simulink model "mpc_lateralcontrol"  (R2021a)
settings: Solver=VariableStepAuto  StartTime=0.0  StopTime=Ts  FixedStep=0.1  RelTol=1e-3
InitFcn:
  | mpc_init
StopFcn:
  | simulation_plots_mpc
values from neighbouring files (symbols this model uses):
  Vx = 25    [mpc_init.m]
libraries: mpclib x1
settings Model: Creator=anime  LastModifiedBy=User
settings SolverCC: AlgebraicLoopSolver=TrustRegion
settings DebuggingCC: SFMachineParentedDataDiag=warning

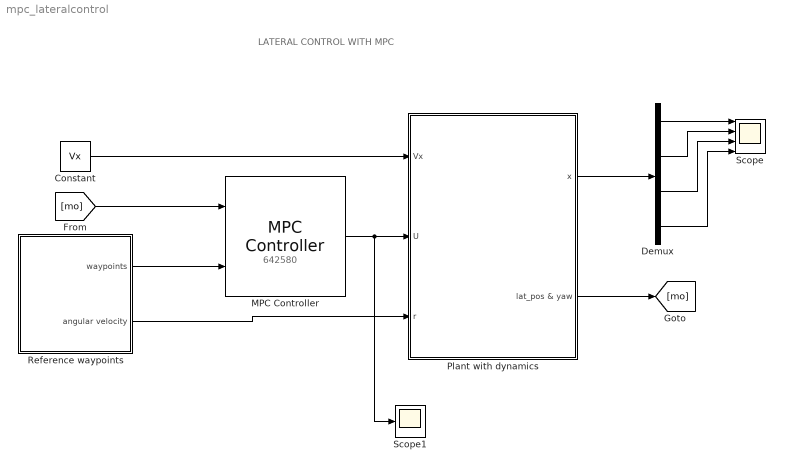
== system mpc_lateralcontrol ==
  note: 642580
  note: LATERAL CONTROL WITH MPC
  Constant : Constant  Value=Vx
  Demux : Demux
  MPC Controller : mpclib/MPC Controller  SCDEnableBlockLinearizationSpecification=on  mpcobj=mpc1  is_multiple=0  enable_value=0  return_u0=off  updateMPCinCallerWorkspace=on  md_inport=off  mv_inport=off  uref_inport=off  return_cost=off  return_mvseq=off  return_qpstatus=off  return_xseq=off  return_state=off  return_ovseq=off  state_inport=off  umin_inport=off  umax_inport=off  ymin_inport=off  ymax_inport=off  cc_inport=off  ywt_inport=off  uwt_inport=off  duwt_inport=off  rhoeps_inport=off  pm_inport=off  MaximumP=10  HorizonChoice=FixedHorizon  n_ts=0.1  n_p=10  n_mv=1  n_md=0  n_ud=0  n_mo=2  n_uo=0  BlockDataType=double  SampleTimeInherited=off  switch_inport=off
  Plant with dynamics : Subsystem
  Reference waypoints : Subsystem
  Scope : Scope  NumInputPorts=4
  Scope1 : Scope
  wires:
  Demux/1 -> Scope/1
  Demux/4 -> Scope/4
  Demux/3 -> Scope/3
  Demux/2 -> Scope/2
  Plant with dynamics/2(lat_pos & yaw) -> [mo]
  Constant/1 -> Plant with dynamics/1(Vx)
  Reference waypoints/2(angular velocity) -> Plant with dynamics/3(r)
  MPC Controller/1 -> Scope1/1, Plant with dynamics/2(U)
  [mo] -> MPC Controller/1
  Reference waypoints/1(waypoints) -> MPC Controller/2
  Plant with dynamics/1(x) -> Demux/1

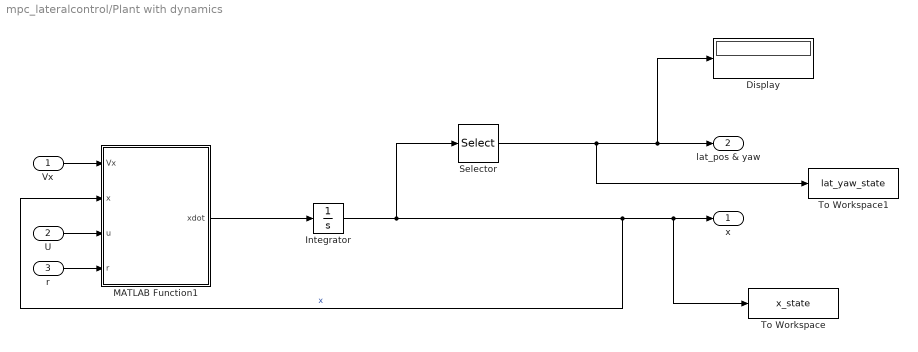
== system mpc_lateralcontrol/Plant with dynamics ==
  Vx : Inport
  U : Inport  Port=2
  r : Inport  Port=3
  Display : Display
  Integrator : Integrator
  MATLAB Function1 : MATLAB Function  TreatAsAtomicUnit=on
  Selector : Selector  InputPortWidth=4  IndexOptions=Index vector (dialog)  Indices=[1 3]  OutputSizes=1
  To Workspace : ToWorkspace  VariableName=x_state  SampleTime=-1
  To Workspace1 : ToWorkspace  VariableName=lat_yaw_state  SampleTime=-1
  x : Outport
  lat_pos & yaw : Outport  Port=2
  wires:
  Vx/1 -> MATLAB Function1/1(Vx)
  U/1 -> MATLAB Function1/3(u)
  r/1 -> MATLAB Function1/4(r)
  Integrator/1 -> Selector/1, MATLAB Function1/2(x), To Workspace/1, x/1  "x"
  Selector/1 -> To Workspace1/1, Display/1, lat_pos & yaw/1
  MATLAB Function1/1(xdot) -> Integrator/1

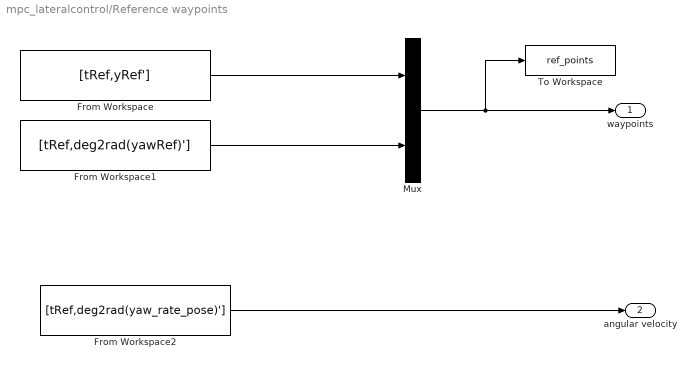
== system mpc_lateralcontrol/Reference waypoints ==
  From Workspace : FromWorkspace  VariableName=[tRef,yRef']  SampleTime=0.1
  From Workspace1 : FromWorkspace  VariableName=[tRef,deg2rad(yawRef)']  SampleTime=0.1
  From Workspace2 : FromWorkspace  VariableName=[tRef,deg2rad(yaw_rate_pose)']  SampleTime=0.1
  Mux : Mux  Inputs=2
  To Workspace : ToWorkspace  VariableName=ref_points  SampleTime=-1
  waypoints : Outport
  angular velocity : Outport  Port=2
  wires:
  Mux/1 -> To Workspace/1, waypoints/1
  From Workspace/1 -> Mux/1
  From Workspace1/1 -> Mux/2
  From Workspace2/1 -> angular velocity/1

== matlab function mpc_lateralcontrol/Plant with dynamics/MATLAB Function1 ==
  data: Vx input; x input; u input; xdot output; r input
function xdot = fcn(Vx,x,u,r)

%% Model parameters
m = 1140;
I_z = 1436.24; %kgm2
l_f = 1.165; 
l_r = 1.165;
c_f = 155494.663;
c_r = 1554494.663;

% assuming constant velocity
v_x = Vx; %mps
%% Dynamic bicycle model 
%continous A B C D matrixes
A = [0 1 0 0;
     0 -2*(c_f+c_r)/(m*v_x) 0 -2*(l_f*c_f + l_r*c_r)/(m*v_x) - v_x;
     0 0 0 1;
     0 2*(l_r*c_r - l_f*c_f)/(I_z*v_x)  0  -2*(l_r^2*c_r - l_f^2*c_f)/(I_z*v_x)];
 
B = [0;
    2*c_f/m;
    0;
    2*l_f*c_f/I_z];
C= [1 0 0 0;
       0 1 0 0];
D = [0;0];

xdot = A*x + B*u;
end
